simulink model "tau_12"  (R2019b)
settings: Solver=VariableStepAuto  StartTime=0.0  StopTime=100  RelTol=1e-3
libraries: simulink x2, slctrlblks x1
settings Model: Creator=Sergey  LastModifiedBy=Sergey

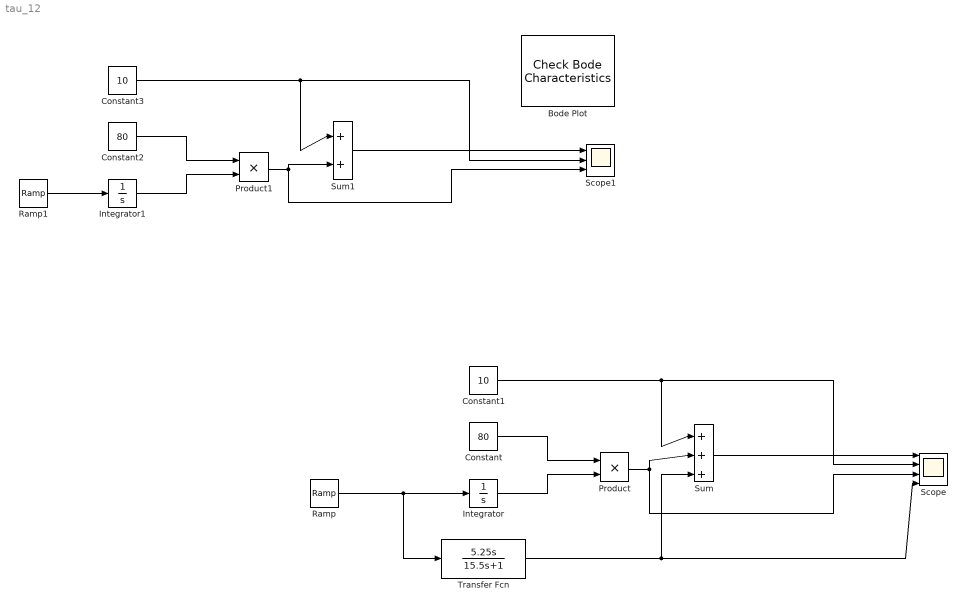
== system tau_12 ==
  Bode Plot : slctrlblks/Model Verification/Check Bode  Characteristics  InstantiateOnLoad=on  SaveOperatingPoints=off  LinearizationIOs={'/Ramp1', 1, 'in', 'off', '';'/Sum1', 1, 'out', 'off', ''}  LinearizeAt=SnapshotTimes  SnapshotTimes=[0]  TriggerType=rising  SampleTime=auto  RateConversionMethod=zoh  PreWarpFreq=10  UseExactDelayModel=off  UseFullBlockNameLabels=off  UseBusSignalLabels=off  enabled=on  stopWhenAssertionFail=off  export=off  ViewDlgPos=[1 41 1920 963]  OpenViewOnLoad=off  LaunchViewOnOpen=on  FrequencyUnits=rad/s  MagnitudeUnits=dB  PhaseUnits=deg  TimeUnits=seconds  EnableUpperBound=off  UpperBoundFrequencies=[]  UpperBoundMagnitudes=[]  EnableLowerBound=off  LowerBoundFrequencies=[]  LowerBoundMagnitudes=[]
      settings: SourceProductName=Simulink Control Design
  Constant : Constant  Value=80
  Constant1 : Constant  Value=10
  Constant2 : Constant  Value=80
  Constant3 : Constant  Value=10
  Integrator : Integrator
  Integrator1 : Integrator
  Product : Product
  Product1 : Product
  Ramp : simulink/Sources/Ramp  slope=1  start=0  InitialOutput=0
  Ramp1 : simulink/Sources/Ramp  slope=1  start=0  InitialOutput=0
  Scope : Scope  NumInputPorts=4
  Scope1 : Scope  NumInputPorts=3
  Sum : Sum  Inputs=|+++
  Sum1 : Sum  Inputs=|++
  Transfer Fcn : TransferFcn  Numerator=[5.25 0]  Denominator=[15.5 1]
  wires:
  Constant/1 -> Product/1
  Integrator/1 -> Product/2
  Ramp/1 -> Transfer Fcn/1, Integrator/1
  Product/1 -> Scope/3, Sum/2
  Constant1/1 -> Scope/2, Sum/1
  Transfer Fcn/1 -> Sum/3, Scope/4
  Sum/1 -> Scope/1
  Sum1/1 -> Scope1/1
  Constant3/1 -> Scope1/2, Sum1/1
  Product1/1 -> Scope1/3, Sum1/2
  Ramp1/1 -> Integrator1/1
  Integrator1/1 -> Product1/2
  Constant2/1 -> Product1/1
